simulink model "MultiInverter_Transient_Simulation_GFM_Load"  (R2020b)
settings: Solver=FixedStepAuto  StartTime=0  StopTime=6  FixedStep=Ts  RelTol=1e-3
undefined symbols (not defined in the file): DeviceDiscreDamping, DevicePara, DevicePowerFlow, DeviceType, Fbase, OtherInputs, Sbase, Ts, Vbase, Wbase, x_e, Ybase, Zbase
libraries: powerlib x61, SimplexPS x24, SimplexPS_ x1
settings Model: Creator=admin_user  LastModifiedBy=admin_user
settings DataIOCC: ReturnWorkspaceOutputs=off

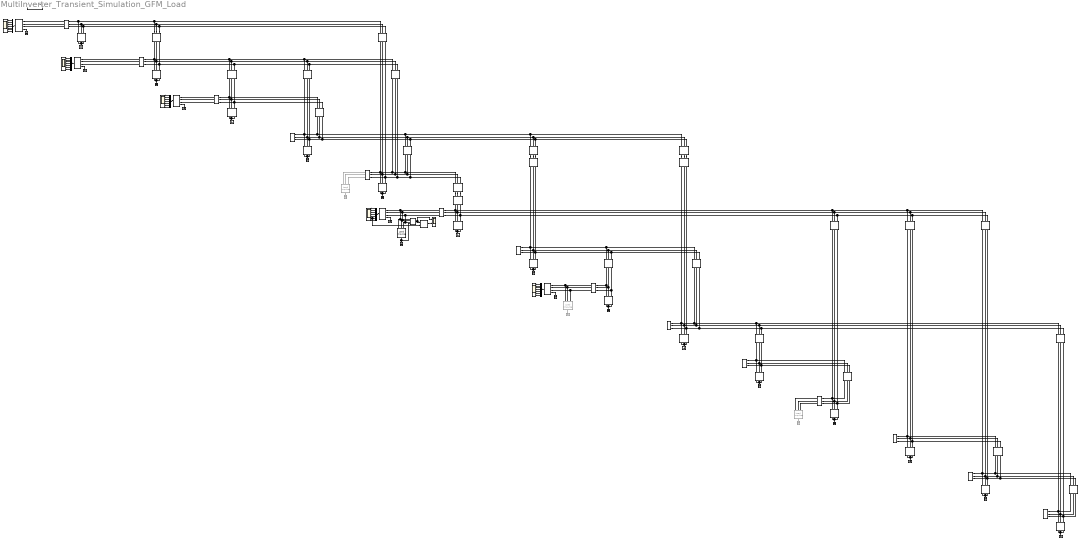
== system MultiInverter_Transient_Simulation_GFM_Load ==
  note: Fault
  note: Fault
  note: Fault
  note: Fault
  B-GND{1,4..5,8,10,14,16,20,23..24,27,29..30,32,34} (15 alike) : powerlib/Elements/Ground  LConnTagsString=a
  B-GND2 : powerlib/Elements/Ground  Commented=on  LConnTagsString=a
  B-GND3 : powerlib/Elements/Ground  Commented=on  LConnTagsString=a
  B-GND6 : powerlib/Elements/Ground  Commented=on  LConnTagsString=a
  Branch1-1 : powerlib/Elements/Three-Phase Parallel RLC Branch  LConnTagsString=A|B|C  RConnTagsString=A|B|C  BranchType=RC  Resistance=(0.5618)*Zbase  Inductance=1e-3  Capacitance=(0.051)*Ybase/Wbase  Measurements=None
      settings: SourceProductBaseCode=PS
  Branch1-2 : powerlib/Elements/Three-Phase Series RLC Branch  LConnTagsString=A|B|C  RConnTagsString=A|B|C  BranchType=RL  Resistance=(0.01938)*Zbase  Inductance=(0.05917)*Zbase/Wbase  Capacitance=1e-6  Measurements=None
  Branch1-5 : powerlib/Elements/Three-Phase Series RLC Branch  LConnTagsString=A|B|C  RConnTagsString=A|B|C  BranchType=RL  Resistance=(0.05403)*Zbase  Inductance=(0.22304)*Zbase/Wbase  Capacitance=1e-6  Measurements=None
  Branch10-10 : powerlib/Elements/Three-Phase Parallel RLC Branch  LConnTagsString=A|B|C  RConnTagsString=A|B|C  BranchType=RL  Resistance=(11.6029)*Zbase  Inductance=(18.0044)*Zbase/Wbase  Capacitance=(0)*Ybase/Wbase  Measurements=None
      settings: SourceProductBaseCode=PS
  Branch10-11 : powerlib/Elements/Three-Phase Series RLC Branch  LConnTagsString=A|B|C  RConnTagsString=A|B|C  BranchType=RL  Resistance=(0.08205)*Zbase  Inductance=(0.19207)*Zbase/Wbase  Capacitance=1e-6  Measurements=None
  Branch11-11 : powerlib/Elements/Three-Phase Parallel RLC Branch  LConnTagsString=A|B|C  RConnTagsString=A|B|C  BranchType=RL  Resistance=(30.7309)*Zbase  Inductance=(59.7546)*Zbase/Wbase  Capacitance=(0)*Ybase/Wbase  Measurements=None
      settings: SourceProductBaseCode=PS
  Branch12-12 : powerlib/Elements/Three-Phase Parallel RLC Branch  LConnTagsString=A|B|C  RConnTagsString=A|B|C  BranchType=RL  Resistance=(17.8442)*Zbase  Inductance=(68.0311)*Zbase/Wbase  Capacitance=(0)*Ybase/Wbase  Measurements=None
      settings: SourceProductBaseCode=PS
  Branch12-13 : powerlib/Elements/Three-Phase Series RLC Branch  LConnTagsString=A|B|C  RConnTagsString=A|B|C  BranchType=RL  Resistance=(0.22092)*Zbase  Inductance=(0.19988)*Zbase/Wbase  Capacitance=1e-6  Measurements=None
  Branch13-13 : powerlib/Elements/Three-Phase Parallel RLC Branch  LConnTagsString=A|B|C  RConnTagsString=A|B|C  BranchType=RL  Resistance=(7.9629)*Zbase  Inductance=(18.5344)*Zbase/Wbase  Capacitance=(0)*Ybase/Wbase  Measurements=None
      settings: SourceProductBaseCode=PS
  Branch13-14 : powerlib/Elements/Three-Phase Series RLC Branch  LConnTagsString=A|B|C  RConnTagsString=A|B|C  BranchType=RL  Resistance=(0.17093)*Zbase  Inductance=(0.34802)*Zbase/Wbase  Capacitance=1e-6  Measurements=None
  Branch14-14 : powerlib/Elements/Three-Phase Parallel RLC Branch  LConnTagsString=A|B|C  RConnTagsString=A|B|C  BranchType=RL  Resistance=(6.8542)*Zbase  Inductance=(20.4256)*Zbase/Wbase  Capacitance=(0)*Ybase/Wbase  Measurements=None
      settings: SourceProductBaseCode=PS
  Branch2-2 : powerlib/Elements/Three-Phase Parallel RLC Branch  LConnTagsString=A|B|C  RConnTagsString=A|B|C  BranchType=RLC  Resistance=(5.0324)*Zbase  Inductance=(8.5986)*Zbase/Wbase  Capacitance=(0.0826)*Ybase/Wbase  Measurements=None
      settings: SourceProductBaseCode=PS
  Branch2-3 : powerlib/Elements/Three-Phase Series RLC Branch  LConnTagsString=A|B|C  RConnTagsString=A|B|C  BranchType=RL  Resistance=(0.04699)*Zbase  Inductance=(0.19797)*Zbase/Wbase  Capacitance=1e-6  Measurements=None
  Branch2-4 : powerlib/Elements/Three-Phase Series RLC Branch  LConnTagsString=A|B|C  RConnTagsString=A|B|C  BranchType=RL  Resistance=(0.05811)*Zbase  Inductance=(0.17632)*Zbase/Wbase  Capacitance=1e-6  Measurements=None
  Branch2-5 : powerlib/Elements/Three-Phase Series RLC Branch  LConnTagsString=A|B|C  RConnTagsString=A|B|C  BranchType=RL  Resistance=(0.05695)*Zbase  Inductance=(0.17388)*Zbase/Wbase  Capacitance=1e-6  Measurements=None
  Branch3-3 : powerlib/Elements/Three-Phase Parallel RLC Branch  LConnTagsString=A|B|C  RConnTagsString=A|B|C  BranchType=RLC  Resistance=(0.34674)*Zbase  Inductance=(5.3689)*Zbase/Wbase  Capacitance=(0.0283)*Ybase/Wbase  Measurements=None
      settings: SourceProductBaseCode=PS
  Branch3-4 : powerlib/Elements/Three-Phase Series RLC Branch  LConnTagsString=A|B|C  RConnTagsString=A|B|C  BranchType=RL  Resistance=(0.06701)*Zbase  Inductance=(0.17103)*Zbase/Wbase  Capacitance=1e-6  Measurements=None
  Branch4-4 : powerlib/Elements/Three-Phase Parallel RLC Branch  LConnTagsString=A|B|C  RConnTagsString=A|B|C  BranchType=RC  Resistance=(2.1492)*Zbase  Inductance=1e-3  Capacitance=(0.061362)*Ybase/Wbase  Measurements=None
      settings: SourceProductBaseCode=PS
  Branch4-5 : powerlib/Elements/Three-Phase Series RLC Branch  LConnTagsString=A|B|C  RConnTagsString=A|B|C  BranchType=RL  Resistance=(0.01335)*Zbase  Inductance=(0.04211)*Zbase/Wbase  Capacitance=1e-6  Measurements=None
  Branch4-7 : powerlib/Elements/Three-Phase Series RLC Branch  LConnTagsString=A|B|C  RConnTagsString=A|B|C  BranchType=RL  Resistance=(0.020912*2)*Zbase  Inductance=(0.20912)*Zbase/Wbase  Capacitance=1e-6  Measurements=None
  Branch4-9 : powerlib/Elements/Three-Phase Series RLC Branch  LConnTagsString=A|B|C  RConnTagsString=A|B|C  BranchType=RL  Resistance=(0.055618*2)*Zbase  Inductance=(0.55618)*Zbase/Wbase  Capacitance=1e-6  Measurements=None
  Branch5-5 : powerlib/Elements/Three-Phase Parallel RLC Branch  LConnTagsString=A|B|C  RConnTagsString=A|B|C  BranchType=RLC  Resistance=(13.6052)*Zbase  Inductance=(64.6247)*Zbase/Wbase  Capacitance=(0.0419)*Ybase/Wbase  Measurements=None
      settings: SourceProductBaseCode=PS
  Branch5-6 : powerlib/Elements/Three-Phase Series RLC Branch  LConnTagsString=A|B|C  RConnTagsString=A|B|C  BranchType=RL  Resistance=(0.025202*2)*Zbase  Inductance=(0.25202)*Zbase/Wbase  Capacitance=1e-6  Measurements=None
  Branch6-11 : powerlib/Elements/Three-Phase Series RLC Branch  LConnTagsString=A|B|C  RConnTagsString=A|B|C  BranchType=RL  Resistance=(0.09498)*Zbase  Inductance=(0.1989)*Zbase/Wbase  Capacitance=1e-6  Measurements=None
  Branch6-12 : powerlib/Elements/Three-Phase Series RLC Branch  LConnTagsString=A|B|C  RConnTagsString=A|B|C  BranchType=RL  Resistance=(0.12291)*Zbase  Inductance=(0.25581)*Zbase/Wbase  Capacitance=1e-6  Measurements=None
  Branch6-13 : powerlib/Elements/Three-Phase Series RLC Branch  LConnTagsString=A|B|C  RConnTagsString=A|B|C  BranchType=RL  Resistance=(0.06615)*Zbase  Inductance=(0.13027)*Zbase/Wbase  Capacitance=1e-6  Measurements=None
  Branch6-6 : powerlib/Elements/Three-Phase Parallel RLC Branch  LConnTagsString=A|B|C  RConnTagsString=A|B|C  BranchType=RL  Resistance=(0.52202)*Zbase  Inductance=(14.9813)*Zbase/Wbase  Capacitance=(0)*Ybase/Wbase  Measurements=None
      settings: SourceProductBaseCode=PS
  Branch7-7 : powerlib/Elements/Three-Phase Parallel RLC Branch  LConnTagsString=A|B|C  RConnTagsString=A|B|C  BranchType=C  Resistance=(Inf)*Zbase  Inductance=1e-3  Capacitance=(0.0005)*Ybase/Wbase  Measurements=None
      settings: SourceProductBaseCode=PS
  Branch7-8 : powerlib/Elements/Three-Phase Series RLC Branch  LConnTagsString=A|B|C  RConnTagsString=A|B|C  BranchType=RL  Resistance=(0.017615*2)*Zbase  Inductance=(0.17615)*Zbase/Wbase  Capacitance=1e-6  Measurements=None
  Branch7-9 : powerlib/Elements/Three-Phase Series RLC Branch  LConnTagsString=A|B|C  RConnTagsString=A|B|C  BranchType=RL  Resistance=(0.011001*2)*Zbase  Inductance=(0.11001)*Zbase/Wbase  Capacitance=1e-6  Measurements=None
  Branch8-8 : powerlib/Elements/Three-Phase Parallel RLC Branch  LConnTagsString=A|B|C  RConnTagsString=A|B|C  BranchType=C  Resistance=(Inf)*Zbase  Inductance=1e-3  Capacitance=(0.0005)*Ybase/Wbase  Measurements=None
      settings: SourceProductBaseCode=PS
  Branch9-10 : powerlib/Elements/Three-Phase Series RLC Branch  LConnTagsString=A|B|C  RConnTagsString=A|B|C  BranchType=RL  Resistance=(0.03181)*Zbase  Inductance=(0.0845)*Zbase/Wbase  Capacitance=1e-6  Measurements=None
  Branch9-14 : powerlib/Elements/Three-Phase Series RLC Branch  LConnTagsString=A|B|C  RConnTagsString=A|B|C  BranchType=RL  Resistance=(0.12711)*Zbase  Inductance=(0.27038)*Zbase/Wbase  Capacitance=1e-6  Measurements=None
  Branch9-9 : powerlib/Elements/Three-Phase Parallel RLC Branch  LConnTagsString=A|B|C  RConnTagsString=A|B|C  BranchType=RL  Resistance=(3.5475)*Zbase  Inductance=(6.3043)*Zbase/Wbase  Capacitance=(0)*Ybase/Wbase  Measurements=None
      settings: SourceProductBaseCode=PS
  Bus{1..14} (14 alike) : SimplexPS/Three-Phase Bus  Vbase=1  Sbase=1
      settings: SourceProductName=Simplex Power Systems
  D-GND{1..3,6,8} (5 alike) : powerlib/Elements/Ground  LConnTagsString=a
  D-Scope{1..3,6,8} (5 alike) : Scope  NumInputPorts=7
  DS-Bus{1..3,6,8} (5 alike) : BusSelector  OutputSignals=v_dq,i_dq,v_abc,i_abc,w,theta,pq
  Load Impulse : SimplexPS/Load Impulse  Commented=on  t0=3  dt=1/50*4  R=1e-20*Zbase
      settings: SourceProductName=Simplex Power Systems
  Load Impulse1 : SimplexPS/Load Impulse  Commented=on  t0=2  dt=1/50*3  R=1e-9*Zbase
      settings: SourceProductName=Simplex Power Systems
  Load Impulse2 : SimplexPS/Load Impulse  t0=5  dt=1/50*3  R=1e-9*Zbase
      settings: SourceProductName=Simplex Power Systems
  Load Impulse3 : SimplexPS/Load Impulse  Commented=on  t0=2  dt=1/50*4  R=1e-9*Zbase
      settings: SourceProductName=Simplex Power Systems
  Scope Voltage : Scope  NumInputPorts=2
  Transformer4-7 : powerlib/Elements/Three-Phase Transformer (Two Windings)  Winding1Connection=Yg  Winding2Connection=Yg  CoreType=Three single-phase transformers  SetSaturation=off  Hysteresis=off  DataFile='hysteresis'  SetInitialFlux=off  Measurements=None  UNITS=pu  NominalPower=[Sbase, Fbase]  Winding1=[0.978*Vbase, 0, 0]  Winding2=[Vbase, 0, 0]  Rm=1e4  Lm=1e4  L0=0.5  Saturation=[ 0,0 ; 0.0024,1.2 ; 1.0,1.52 ]  InitialFluxes=[ 0.8 , -0.8 , 0.7 ]  BreakLoop=off  DiscreteSolver=Trapezoidal iterative  DataType=off  TransfoNumber=1
  Transformer4-9 : powerlib/Elements/Three-Phase Transformer (Two Windings)  Winding1Connection=Yg  Winding2Connection=Yg  CoreType=Three single-phase transformers  SetSaturation=off  Hysteresis=off  DataFile='hysteresis'  SetInitialFlux=off  Measurements=None  UNITS=pu  NominalPower=[Sbase, Fbase]  Winding1=[0.969*Vbase, 0, 0]  Winding2=[Vbase, 0, 0]  Rm=1e4  Lm=1e4  L0=0.5  Saturation=[ 0,0 ; 0.0024,1.2 ; 1.0,1.52 ]  InitialFluxes=[ 0.8 , -0.8 , 0.7 ]  BreakLoop=off  DiscreteSolver=Trapezoidal iterative  DataType=off  TransfoNumber=1
  Transformer5-6 : powerlib/Elements/Three-Phase Transformer (Two Windings)  Winding1Connection=Yg  Winding2Connection=Yg  CoreType=Three single-phase transformers  SetSaturation=off  Hysteresis=off  DataFile='hysteresis'  SetInitialFlux=off  Measurements=None  UNITS=pu  NominalPower=[Sbase, Fbase]  Winding1=[0.932*Vbase, 0, 0]  Winding2=[Vbase, 0, 0]  Rm=1e4  Lm=1e4  L0=0.5  Saturation=[ 0,0 ; 0.0024,1.2 ; 1.0,1.52 ]  InitialFluxes=[ 0.8 , -0.8 , 0.7 ]  BreakLoop=off  DiscreteSolver=Trapezoidal iterative  DataType=off  TransfoNumber=1
  VSI-Droop1 : SimplexPS/Grid-Forming Voltage-Source Inverter (dq-Frame System Object)  Ts=Ts  Sbase=Sbase  Vbase=Vbase  Wbase=Wbase  DeviceType=DeviceType{1}  DevicePara=DevicePara{1}  PowerFlow=DevicePowerFlow{1}  x0=x_e{1}  OtherInputs=OtherInputs{1}  DiscreMethod=Hybrid Trapezoidal  EnableInsideModification=off  DiscreDampingFlag=on  DiscreDampingValue=DeviceDiscreDamping{1}  LinearizationTimes=1  DirectFeedthrough=off
      settings: SourceProductName=Simplex Power Systems
  VSI-Droop3 : SimplexPS/Grid-Forming Voltage-Source Inverter (dq-Frame System Object)  Ts=Ts  Sbase=Sbase  Vbase=Vbase  Wbase=Wbase  DeviceType=DeviceType{3}  DevicePara=DevicePara{3}  PowerFlow=DevicePowerFlow{3}  x0=x_e{3}  OtherInputs=OtherInputs{3}  DiscreMethod=Hybrid Trapezoidal  EnableInsideModification=off  DiscreDampingFlag=on  DiscreDampingValue=DeviceDiscreDamping{3}  LinearizationTimes=1  DirectFeedthrough=off
      settings: SourceProductName=Simplex Power Systems
  VSI-Droop6 : SimplexPS/Grid-Forming Voltage-Source Inverter (dq-Frame System Object)  Ts=Ts  Sbase=Sbase  Vbase=Vbase  Wbase=Wbase  DeviceType=DeviceType{6}  DevicePara=DevicePara{6}  PowerFlow=DevicePowerFlow{6}  x0=x_e{6}  OtherInputs=OtherInputs{6}  DiscreMethod=Hybrid Trapezoidal  EnableInsideModification=off  DiscreDampingFlag=on  DiscreDampingValue=DeviceDiscreDamping{6}  LinearizationTimes=1  DirectFeedthrough=off
      settings: SourceProductName=Simplex Power Systems
  VSI-PLL2 : SimplexPS/Grid-Following Voltage-Source Inverter (dq-Frame System Object)  Ts=Ts  Sbase=Sbase  Vbase=Vbase  Wbase=Wbase  DeviceType=DeviceType{2}  DevicePara=DevicePara{2}  PowerFlow=DevicePowerFlow{2}  x0=x_e{2}  OtherInputs=OtherInputs{2}  DiscreMethod=Hybrid Trapezoidal  EnableInsideModification=off  DiscreDampingFlag=on  DiscreDampingValue=DeviceDiscreDamping{2}  LinearizationTimes=1  DirectFeedthrough=off
      settings: SourceProductName=Simplex Power Systems
  VSI-PLL8 : SimplexPS/Grid-Following Voltage-Source Inverter (dq-Frame System Object)  Ts=Ts  Sbase=Sbase  Vbase=Vbase  Wbase=Wbase  DeviceType=DeviceType{8}  DevicePara=DevicePara{8}  PowerFlow=DevicePowerFlow{8}  x0=x_e{8}  OtherInputs=OtherInputs{8}  DiscreMethod=Hybrid Trapezoidal  EnableInsideModification=off  DiscreDampingFlag=on  DiscreDampingValue=DeviceDiscreDamping{8}  LinearizationTimes=1  DirectFeedthrough=off
      settings: SourceProductName=Simplex Power Systems
  "Voltage Measurement (3ph -> 3ph)" : SimplexPS/Voltage Measurement (3ph -> 3ph)  SystemSampleTime=-1  VariantActivationTime=update diagram  Latency=0  AutoFrameSizeCalculation=off
      settings: SourceProductName=Simplex Power Systems
  "abc -> dq (Power-Invariant)1" : SimplexPS_/abc -> dq (Power-Invariant)  SystemSampleTime=-1  VariantActivationTime=update diagram  Latency=0  AutoFrameSizeCalculation=off
  powergui : powerlib/powergui  Priority=1  SimulationMode=Discrete  SampleTime=Ts  frequency=60  Iterations=50  frequencyindice=0  Pbase=100e6  ErrMax=1e-4  UnitsV=kV  UnitsW=MW  buscounter=0  FunctionMessages=off  echomessages=off  EnableUseOfTLC=off  CurrentSourceSwitches=off  DisableSnubberDevices=off  DisableRonSwitches=off  DisableVfSwitches=off  DisplayEquations=off  AutomaticDiscreteSolvers=off  SolverType=Tustin/Backward Euler (TBE)  Interpol=off  ExternalGateDelay=off  methode=off  Ts=100  x0status=blocks  SPID=on  SwTol=0  HookPort=off  NonlinearTolerance=1e-4  nMaxIteration=100  ContinueOnMaxIteration=off  RestoreLinks=warning  ResistiveCurrentMeasurement=off  Frange=[0:2:500]  Ylog=off  Xlog=on  ShowGrid=off  save=off  variable=ZData  structure=0  ZoomFFT=off  StartTime=0.0  cycles=1  DisplayStyle=1  fundamental=60  FreqAxis=off  MaxFrequency=1000  frequencyindicesteady=1  RmsSteady=1  display=off
  wires:
  VSI-Droop1/1 -> DS-Bus1/1
  DS-Bus1/1 -> D-Scope1/1  "<v_dq>"
  DS-Bus1/2 -> D-Scope1/2  "<i_dq>"
  DS-Bus1/3 -> D-Scope1/3  "<v_abc>"
  DS-Bus1/4 -> D-Scope1/4  "<i_abc>"
  DS-Bus1/5 -> D-Scope1/5  "<w>"
  DS-Bus1/6 -> D-Scope1/6  "<theta>"
  DS-Bus1/7 -> D-Scope1/7  "<pq>"
  VSI-PLL2/1 -> DS-Bus2/1
  DS-Bus2/1 -> D-Scope2/1  "<v_dq>"
  DS-Bus2/2 -> D-Scope2/2  "<i_dq>"
  DS-Bus2/3 -> D-Scope2/3  "<v_abc>"
  DS-Bus2/4 -> D-Scope2/4  "<i_abc>"
  DS-Bus2/5 -> D-Scope2/5  "<w>"
  DS-Bus2/6 -> D-Scope2/6  "<theta>"
  DS-Bus2/7 -> D-Scope2/7  "<pq>"
  VSI-Droop3/1 -> DS-Bus3/1
  DS-Bus3/1 -> D-Scope3/1  "<v_dq>"
  DS-Bus3/2 -> D-Scope3/2  "<i_dq>"
  DS-Bus3/3 -> D-Scope3/3  "<v_abc>"
  DS-Bus3/4 -> D-Scope3/4  "<i_abc>"
  DS-Bus3/5 -> D-Scope3/5  "<w>"
  DS-Bus3/6 -> D-Scope3/6  "<theta>"
  DS-Bus3/7 -> D-Scope3/7  "<pq>"
  VSI-Droop6/1 -> DS-Bus6/1
  DS-Bus6/1 -> D-Scope6/1  "<v_dq>"
  DS-Bus6/2 -> D-Scope6/2  "<i_dq>"
  DS-Bus6/3 -> D-Scope6/3  "<v_abc>"
  DS-Bus6/4 -> D-Scope6/4  "<i_abc>"
  DS-Bus6/5 -> D-Scope6/5  "<w>"
  DS-Bus6/6 -> "abc -> dq (Power-Invariant)1"/2, D-Scope6/6  "<theta>"
  DS-Bus6/7 -> D-Scope6/7  "<pq>"
  VSI-PLL8/1 -> DS-Bus8/1
  DS-Bus8/1 -> D-Scope8/1  "<v_dq>"
  DS-Bus8/2 -> D-Scope8/2  "<i_dq>"
  DS-Bus8/3 -> D-Scope8/3  "<v_abc>"
  DS-Bus8/4 -> D-Scope8/4  "<i_abc>"
  DS-Bus8/5 -> D-Scope8/5  "<w>"
  DS-Bus8/6 -> D-Scope8/6  "<theta>"
  DS-Bus8/7 -> D-Scope8/7  "<pq>"
  "Voltage Measurement (3ph -> 3ph)"/1 -> Scope Voltage/1, "abc -> dq (Power-Invariant)1"/1
  "abc -> dq (Power-Invariant)1"/1 -> Scope Voltage/2
  connections:
  VSI-Droop1/LConn4 -- D-GND1/LConn1
  VSI-PLL2/LConn4 -- D-GND2/LConn1
  VSI-Droop3/LConn4 -- D-GND3/LConn1
  VSI-Droop6/LConn4 -- D-GND6/LConn1
  VSI-PLL8/LConn4 -- D-GND8/LConn1
  Branch1-1/RConn1 -- Branch1-1/RConn2 -- Branch1-1/RConn3 -- B-GND1/LConn1
  Branch2-2/RConn1 -- Branch2-2/RConn2 -- Branch2-2/RConn3 -- B-GND4/LConn1
  Branch3-3/RConn1 -- Branch3-3/RConn2 -- Branch3-3/RConn3 -- B-GND8/LConn1
  Branch4-4/RConn1 -- Branch4-4/RConn2 -- Branch4-4/RConn3 -- B-GND10/LConn1
  Branch5-5/RConn1 -- Branch5-5/RConn2 -- Branch5-5/RConn3 -- B-GND14/LConn1
  Branch6-6/RConn1 -- Branch6-6/RConn2 -- Branch6-6/RConn3 -- B-GND16/LConn1
  Branch7-7/RConn1 -- Branch7-7/RConn2 -- Branch7-7/RConn3 -- B-GND20/LConn1
  Branch8-8/RConn1 -- Branch8-8/RConn2 -- Branch8-8/RConn3 -- B-GND23/LConn1
  Branch9-9/RConn1 -- Branch9-9/RConn2 -- Branch9-9/RConn3 -- B-GND24/LConn1
  Branch10-10/RConn1 -- Branch10-10/RConn2 -- Branch10-10/RConn3 -- B-GND27/LConn1
  Branch11-11/RConn1 -- Branch11-11/RConn2 -- Branch11-11/RConn3 -- B-GND29/LConn1
  Branch12-12/RConn1 -- Branch12-12/RConn2 -- Branch12-12/RConn3 -- B-GND30/LConn1
  Branch13-13/RConn1 -- Branch13-13/RConn2 -- Branch13-13/RConn3 -- B-GND32/LConn1
  Branch14-14/RConn1 -- Branch14-14/RConn2 -- Branch14-14/RConn3 -- B-GND34/LConn1
  Branch1-2/RConn1 -- Bus2/RConn1 -- Branch2-2/LConn1 -- Branch2-5/LConn1 -- Branch2-4/LConn1 -- Branch2-3/LConn1
  Branch1-2/RConn2 -- Bus2/RConn2 -- Branch2-2/LConn2 -- Branch2-5/LConn2 -- Branch2-4/LConn2 -- Branch2-3/LConn2
  Branch1-2/RConn3 -- Bus2/RConn3 -- Branch2-2/LConn3 -- Branch2-5/LConn3 -- Branch2-4/LConn3 -- Branch2-3/LConn3
  Branch1-2/LConn1 -- Bus1/RConn1 -- Branch1-1/LConn1 -- Branch1-5/LConn1
  Branch1-2/LConn2 -- Bus1/RConn2 -- Branch1-1/LConn2 -- Branch1-5/LConn2
  Branch1-2/LConn3 -- Bus1/RConn3 -- Branch1-1/LConn3 -- Branch1-5/LConn3
  Branch1-5/RConn1 -- Bus5/RConn1 -- Branch5-5/LConn1 -- Transformer5-6/LConn1 -- Branch4-5/RConn1 -- Branch2-5/RConn1
  Branch1-5/RConn2 -- Bus5/RConn2 -- Branch5-5/LConn2 -- Transformer5-6/LConn2 -- Branch4-5/RConn2 -- Branch2-5/RConn2
  Branch1-5/RConn3 -- Bus5/RConn3 -- Branch5-5/LConn3 -- Transformer5-6/LConn3 -- Branch4-5/RConn3 -- Branch2-5/RConn3
  Branch2-3/RConn1 -- Bus3/RConn1 -- Branch3-3/LConn1 -- Branch3-4/LConn1
  Branch2-3/RConn2 -- Bus3/RConn2 -- Branch3-3/LConn2 -- Branch3-4/LConn2
  Branch2-3/RConn3 -- Bus3/RConn3 -- Branch3-3/LConn3 -- Branch3-4/LConn3
  Branch2-4/RConn1 -- Bus4/RConn1 -- Branch4-4/LConn1 -- Transformer4-9/LConn1 -- Transformer4-7/LConn1 -- Branch4-5/LConn1 -- Branch3-4/RConn1
  Branch2-4/RConn2 -- Bus4/RConn2 -- Branch4-4/LConn2 -- Transformer4-9/LConn2 -- Transformer4-7/LConn2 -- Branch4-5/LConn2 -- Branch3-4/RConn2
  Branch2-4/RConn3 -- Bus4/RConn3 -- Branch4-4/LConn3 -- Transformer4-9/LConn3 -- Transformer4-7/LConn3 -- Branch4-5/LConn3 -- Branch3-4/RConn3
  Branch4-7/RConn1 -- Bus7/RConn1 -- Branch7-7/LConn1 -- Branch7-9/LConn1 -- Branch7-8/LConn1
  Branch4-7/RConn2 -- Bus7/RConn2 -- Branch7-7/LConn2 -- Branch7-9/LConn2 -- Branch7-8/LConn2
  Branch4-7/RConn3 -- Bus7/RConn3 -- Branch7-7/LConn3 -- Branch7-9/LConn3 -- Branch7-8/LConn3
  Transformer4-7/RConn1 -- Branch4-7/LConn1
  Transformer4-7/RConn2 -- Branch4-7/LConn2
  Transformer4-7/RConn3 -- Branch4-7/LConn3
  Branch4-9/RConn1 -- Bus9/RConn1 -- Branch9-9/LConn1 -- Branch9-14/LConn1 -- Branch9-10/LConn1 -- Branch7-9/RConn1
  Branch4-9/RConn2 -- Bus9/RConn2 -- Branch9-9/LConn2 -- Branch9-14/LConn2 -- Branch9-10/LConn2 -- Branch7-9/RConn2
  Branch4-9/RConn3 -- Bus9/RConn3 -- Branch9-9/LConn3 -- Branch9-14/LConn3 -- Branch9-10/LConn3 -- Branch7-9/RConn3
  Transformer4-9/RConn1 -- Branch4-9/LConn1
  Transformer4-9/RConn2 -- Branch4-9/LConn2
  Transformer4-9/RConn3 -- Branch4-9/LConn3
  Branch5-6/RConn1 -- Bus6/RConn1 -- Branch6-6/LConn1 -- Branch6-13/LConn1 -- Branch6-12/LConn1 -- Branch6-11/LConn1
  Branch5-6/RConn2 -- Bus6/RConn2 -- Branch6-6/LConn2 -- Branch6-13/LConn2 -- Branch6-12/LConn2 -- Branch6-11/LConn2
  Branch5-6/RConn3 -- Bus6/RConn3 -- Branch6-6/LConn3 -- Branch6-13/LConn3 -- Branch6-12/LConn3 -- Branch6-11/LConn3
  Transformer5-6/RConn1 -- Branch5-6/LConn1
  Transformer5-6/RConn2 -- Branch5-6/LConn2
  Transformer5-6/RConn3 -- Branch5-6/LConn3
  Branch6-11/RConn1 -- Bus11/RConn1 -- Branch11-11/LConn1 -- Branch10-11/RConn1
  Branch6-11/RConn2 -- Bus11/RConn2 -- Branch11-11/LConn2 -- Branch10-11/RConn2
  Branch6-11/RConn3 -- Bus11/RConn3 -- Branch11-11/LConn3 -- Branch10-11/RConn3
  Branch6-12/RConn1 -- Bus12/RConn1 -- Branch12-12/LConn1 -- Branch12-13/LConn1
  Branch6-12/RConn2 -- Bus12/RConn2 -- Branch12-12/LConn2 -- Branch12-13/LConn2
  Branch6-12/RConn3 -- Bus12/RConn3 -- Branch12-12/LConn3 -- Branch12-13/LConn3
  Branch6-13/RConn1 -- Bus13/RConn1 -- Branch13-13/LConn1 -- Branch13-14/LConn1 -- Branch12-13/RConn1
  Branch6-13/RConn2 -- Bus13/RConn2 -- Branch13-13/LConn2 -- Branch13-14/LConn2 -- Branch12-13/RConn2
  Branch6-13/RConn3 -- Bus13/RConn3 -- Branch13-13/LConn3 -- Branch13-14/LConn3 -- Branch12-13/RConn3
  Branch7-8/RConn1 -- Bus8/RConn1 -- Branch8-8/LConn1
  Branch7-8/RConn2 -- Bus8/RConn2 -- Branch8-8/LConn2
  Branch7-8/RConn3 -- Bus8/RConn3 -- Branch8-8/LConn3
  Branch9-10/RConn1 -- Bus10/RConn1 -- Branch10-10/LConn1 -- Branch10-11/LConn1
  Branch9-10/RConn2 -- Bus10/RConn2 -- Branch10-10/LConn2 -- Branch10-11/LConn2
  Branch9-10/RConn3 -- Bus10/RConn3 -- Branch10-10/LConn3 -- Branch10-11/LConn3
  Branch9-14/RConn1 -- Bus14/RConn1 -- Branch14-14/LConn1 -- Branch13-14/RConn1
  Branch9-14/RConn2 -- Bus14/RConn2 -- Branch14-14/LConn2 -- Branch13-14/RConn2
  Branch9-14/RConn3 -- Bus14/RConn3 -- Branch14-14/LConn3 -- Branch13-14/RConn3
  VSI-Droop1/LConn1 -- Bus1/LConn1
  VSI-Droop1/LConn2 -- Bus1/LConn2
  VSI-Droop1/LConn3 -- Bus1/LConn3
  VSI-PLL2/LConn1 -- Bus2/LConn1
  VSI-PLL2/LConn2 -- Bus2/LConn2
  VSI-PLL2/LConn3 -- Bus2/LConn3
  VSI-Droop3/LConn1 -- Bus3/LConn1
  VSI-Droop3/LConn2 -- Bus3/LConn2
  VSI-Droop3/LConn3 -- Bus3/LConn3
  VSI-Droop6/LConn1 -- "Voltage Measurement (3ph -> 3ph)"/LConn1 -- Load Impulse2/LConn1 -- Bus6/LConn1
  VSI-Droop6/LConn2 -- "Voltage Measurement (3ph -> 3ph)"/LConn2 -- Load Impulse2/LConn2 -- Bus6/LConn2
  VSI-Droop6/LConn3 -- "Voltage Measurement (3ph -> 3ph)"/LConn3 -- Load Impulse2/LConn3 -- Bus6/LConn3
  VSI-PLL8/LConn1 -- Load Impulse3/LConn1 -- Bus8/LConn1
  VSI-PLL8/LConn2 -- Bus8/LConn2 -- Load Impulse3/LConn2
  VSI-PLL8/LConn3 -- Bus8/LConn3 -- Load Impulse3/LConn3
  B-GND2/LConn1 -- Load Impulse/RConn1
  Load Impulse/LConn3 -- Bus5/LConn3
  Load Impulse/LConn2 -- Bus5/LConn2
  Load Impulse/LConn1 -- Bus5/LConn1
  Bus11/LConn3 -- Load Impulse1/LConn3
  Bus11/LConn1 -- Load Impulse1/LConn1
  B-GND3/LConn1 -- Load Impulse1/RConn1
  Bus11/LConn2 -- Load Impulse1/LConn2
  B-GND5/LConn1 -- Load Impulse2/RConn1 -- "Voltage Measurement (3ph -> 3ph)"/LConn4
  B-GND6/LConn1 -- Load Impulse3/RConn1
